simulink model "Tra_GearInfo"  (R2016b)
settings: configuration reference "CodeGenConfigSet" (kept outside this file)
values from neighbouring files (symbols this model uses):
  PT_stTraRevGear_C = Calibration.Parameter    [init_Tra_GearInfo.m]    (also in init_Tra_GearInfo_SIL.m = Simulink.Parameter)
  Tra_bStrtStopEnaDfl_C = Calibration.Parameter    [init_Tra_GearInfo.m]    (also in init_Tra_GearInfo_SIL.m = Simulink.Parameter)
  Tra_facN2NPT1_C = Calibration.Parameter    [init_Tra_GearInfo.m]    (also in init_Tra_GearInfo_SIL.m = Simulink.Parameter)
  Tra_facNPT1_C = Calibration.Parameter    [init_Tra_GearInfo.m]    (also in init_Tra_GearInfo_SIL.m = Simulink.Parameter)
  Tra_facV2NPT1_C = Calibration.Parameter    [init_Tra_GearInfo.m]    (also in init_Tra_GearInfo_SIL.m = Simulink.Parameter)
  Tra_GearWide_C = Calibration.Parameter    [init_Tra_GearInfo.m]    (also in init_Tra_GearInfo_SIL.m = Simulink.Parameter)
  Tra_nCrdShMin_C = Calibration.Parameter    [init_Tra_GearInfo.m]    (also in init_Tra_GearInfo_SIL.m = Simulink.Parameter)
  Tra_nEngMin_C = Calibration.Parameter    [init_Tra_GearInfo.m]    (also in init_Tra_GearInfo_SIL.m = Simulink.Parameter)
  Tra_numGearDfl1_C = Calibration.Parameter    [init_Tra_GearInfo.m]    (also in init_Tra_GearInfo_SIL.m = Simulink.Parameter)
  Tra_numGearDfl2_C = Calibration.Parameter    [init_Tra_GearInfo.m]    (also in init_Tra_GearInfo_SIL.m = Simulink.Parameter)
  Tra_numGearTable_CA = Calibration.Parameter    [init_Tra_GearInfo.m]    (also in init_Tra_GearInfo_SIL.m = Simulink.Parameter)
  Tra_rN2NGbxMax_C = Calibration.Parameter    [init_Tra_GearInfo.m]    (also in init_Tra_GearInfo_SIL.m = Simulink.Parameter)
  Tra_rN2NGbxMin_C = Calibration.Parameter    [init_Tra_GearInfo.m]    (also in init_Tra_GearInfo_SIL.m = Simulink.Parameter)
  Tra_rnFacCrdS_C = Calibration.Parameter    [init_Tra_GearInfo.m]    (also in init_Tra_GearInfo_SIL.m = Simulink.Parameter)
  Tra_rTransTable_CA = Calibration.Parameter    [init_Tra_GearInfo.m]    (also in init_Tra_GearInfo_SIL.m = Simulink.Parameter)
  Tra_rV2NDfl_C = Calibration.Parameter    [init_Tra_GearInfo.m]    (also in init_Tra_GearInfo_SIL.m = Simulink.Parameter)
  Tra_rV2NMax_C = Calibration.Parameter    [init_Tra_GearInfo.m]    (also in init_Tra_GearInfo_SIL.m = Simulink.Parameter)
  Tra_rV2NMin_C = Calibration.Parameter    [init_Tra_GearInfo.m]    (also in init_Tra_GearInfo_SIL.m = Simulink.Parameter)
  Tra_SumGear_C = Calibration.Parameter    [init_Tra_GearInfo.m]    (also in init_Tra_GearInfo_SIL.m = Simulink.Parameter)
  Tra_swtSrcCrdSSpdVal_C = Calibration.Parameter    [init_Tra_GearInfo.m]    (also in init_Tra_GearInfo_SIL.m = Simulink.Parameter)
undefined symbols (not defined in the file or in its folder): PT_TraType_State_conv, Switch_conv
libraries: CXLib x5
settings Model: PauseTimes=1  Creator=Colin  LastModifiedBy=bianxuyin
settings ConfigSetRef: SourceLocation=Base Workspace

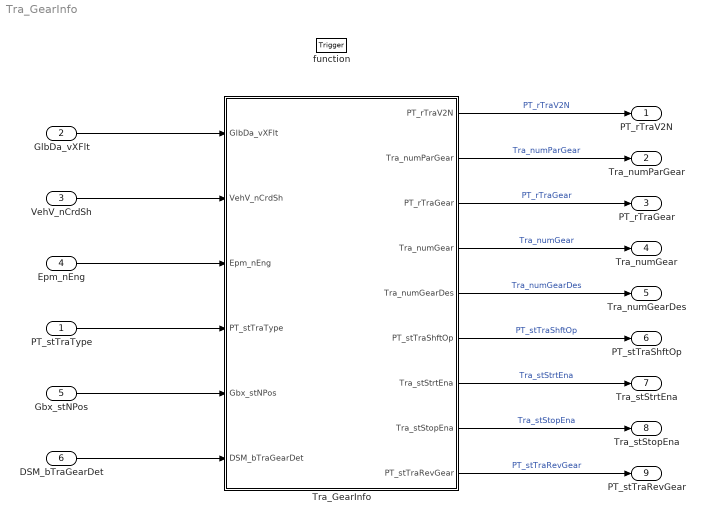
== system Tra_GearInfo ==
  PT_stTraType : Inport  Description=Current transmission type  OutDataTypeStr=Enum: PT_TraType_State_conv
  GlbDa_vXFlt : Inport  Tag=km/h  Description=Vehicle velocity filtered  Port=2  OutMin=0  OutMax=250  OutDataTypeStr=VehSpeed_km_h
  VehV_nCrdSh : Inport  Tag=rpm  Description=Cardan shaft speed  Port=3  OutMin=0  OutMax=6000  OutDataTypeStr=EngSpeed_rpm
  Epm_nEng : Inport  Tag=rpm  Description=Engine speed  Port=4  OutMin=0  OutMax=6000  OutDataTypeStr=EngSpeed_rpm
  Gbx_stNPos : Inport  Description=Gearbox neutral position status signal  Port=5  OutMin=0  OutMax=255  OutDataTypeStr=State_uint8
  DSM_bTraGearDet : Inport  Description=Fault Indicator of Gear Detect Function  Port=6  OutMin=0  OutMax=1  OutDataTypeStr=boolean
  function : TriggerPort  TriggerType=function-call  VariantControl=Variant
  Tra_GearInfo : Subsystem  RTWFcnName=Tra_GearInfo_Co  RTWFileName=Tra_GearInfo
      settings: RTWSystemCode=Nonreusable function  RTWFcnNameOpts=User specified  RTWFileNameOpts=User specified
  PT_rTraV2N : Outport  Tag=km/h/rpm  Description=Quotient of velocity and engine speed  OutMin=-0.32768  OutMax=0.32767  OutDataTypeStr=Tra_V2N_km_h_rpm
  Tra_numParGear : Outport  Description=Application parameter for gear number of the parameter gear of the transmission  Port=2  OutMin=-128  OutMax=127  OutDataTypeStr=Tra_num
  PT_rTraGear : Outport  Description=Current ratio for transmission  Port=3  OutMin=-100  OutMax=100  OutDataTypeStr=TransRatio
  Tra_numGear : Outport  Description=Current gear information  Port=4  OutMin=-128  OutMax=127  OutDataTypeStr=Tra_num
  Tra_numGearDes : Outport  Description=Application parameter for gear number of the destination gear of the transmission  Port=5  OutMin=-128  OutMax=127  OutDataTypeStr=Tra_num
  PT_stTraShftOp : Outport  Description=Status if shift operation is active  Port=6  OutMin=0  OutMax=1  OutDataTypeStr=boolean
  Tra_stStrtEna : Outport  Description=Enable start function  Port=7  OutMin=0  OutMax=1  OutDataTypeStr=boolean
  Tra_stStopEna : Outport  Description=Enable stop function  Port=8  OutMin=0  OutMax=1  OutDataTypeStr=boolean
  PT_stTraRevGear : Outport  Description=Status if reverse gear is selected  Port=9  OutMin=0  OutMax=1  OutDataTypeStr=boolean
  wires:
  Tra_GearInfo/2(Tra_numParGear) -> Tra_numParGear/1  "Tra_numParGear"
  Tra_GearInfo/3(PT_rTraGear) -> PT_rTraGear/1  "PT_rTraGear"
  Tra_GearInfo/4(Tra_numGear) -> Tra_numGear/1  "Tra_numGear"
  Tra_GearInfo/5(Tra_numGearDes) -> Tra_numGearDes/1  "Tra_numGearDes"
  Tra_GearInfo/6(PT_stTraShftOp) -> PT_stTraShftOp/1  "PT_stTraShftOp"
  Tra_GearInfo/7(Tra_stStrtEna) -> Tra_stStrtEna/1  "Tra_stStrtEna"
  Tra_GearInfo/8(Tra_stStopEna) -> Tra_stStopEna/1  "Tra_stStopEna"
  GlbDa_vXFlt/1 -> Tra_GearInfo/1(GlbDa_vXFlt)
  PT_stTraType/1 -> Tra_GearInfo/4(PT_stTraType)
  VehV_nCrdSh/1 -> Tra_GearInfo/2(VehV_nCrdSh)
  Epm_nEng/1 -> Tra_GearInfo/3(Epm_nEng)
  Gbx_stNPos/1 -> Tra_GearInfo/5(Gbx_stNPos)
  Tra_GearInfo/1(PT_rTraV2N) -> PT_rTraV2N/1  "PT_rTraV2N"
  DSM_bTraGearDet/1 -> Tra_GearInfo/6(DSM_bTraGearDet)
  Tra_GearInfo/9(PT_stTraRevGear) -> PT_stTraRevGear/1  "PT_stTraRevGear"

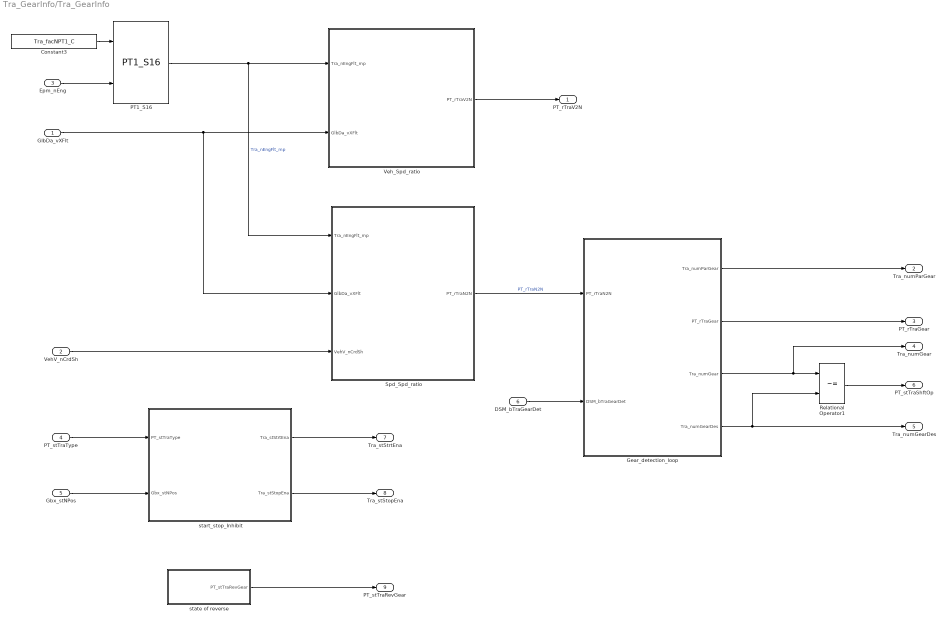
== system Tra_GearInfo/Tra_GearInfo ==
  GlbDa_vXFlt : Inport
  VehV_nCrdSh : Inport  Port=2
  Epm_nEng : Inport  Port=3
  PT_stTraType : Inport  Port=4
  Gbx_stNPos : Inport  Port=5
  DSM_bTraGearDet : Inport  Port=6
  Constant3 : Constant  RequirementInfo={} %GIDa_68e8745b_1911_4ff8_b2e8_39acb6395a61  Value=Tra_facNPT1_C  SampleTime=-1
  Gear_detection_loop : Subsystem
  PT1_S16 : CXLib/PT1_S16
  Relational Operator1 : RelationalOperator  Operator=~=  OutDataTypeStr=boolean  RndMeth=Simplest  InputSameDT=on
  Spd_Spd_ratio : Subsystem
  Veh_Spd_ratio : Subsystem
  start_stop_Inhibit : Subsystem
  state of reverse : Subsystem
  PT_rTraV2N : Outport
  Tra_numParGear : Outport  Port=2
  PT_rTraGear : Outport  Port=3
  Tra_numGear : Outport  Port=4
  Tra_numGearDes : Outport  Port=5
  PT_stTraShftOp : Outport  Port=6
  Tra_stStrtEna : Outport  Port=7
  Tra_stStopEna : Outport  Port=8
  PT_stTraRevGear : Outport  Port=9
  wires:
  Constant3/1 -> PT1_S16/1
  PT1_S16/1 -> Spd_Spd_ratio/1(Tra_nEngFlt_mp), Veh_Spd_ratio/1(Tra_nEngFlt_mp)  "Tra_nEngFlt_mp"
  Epm_nEng/1 -> PT1_S16/2
  Veh_Spd_ratio/1(PT_rTraV2N) -> PT_rTraV2N/1
  VehV_nCrdSh/1 -> Spd_Spd_ratio/3(VehV_nCrdSh)
  GlbDa_vXFlt/1 -> Spd_Spd_ratio/2(GlbDa_vXFlt), Veh_Spd_ratio/2(GlbDa_vXFlt)
  Gear_detection_loop/1(Tra_numParGear) -> Tra_numParGear/1
  Gear_detection_loop/2(PT_rTraGear) -> PT_rTraGear/1
  Gear_detection_loop/4(Tra_numGearDes) -> Relational Operator1/2, Tra_numGearDes/1
  Gear_detection_loop/3(Tra_numGear) -> Tra_numGear/1, Relational Operator1/1
  Spd_Spd_ratio/1(PT_rTraN2N) -> Gear_detection_loop/1(PT_rTraN2N)  "PT_rTraN2N"
  PT_stTraType/1 -> start_stop_Inhibit/1(PT_stTraType)
  Gbx_stNPos/1 -> start_stop_Inhibit/2(Gbx_stNPos)
  start_stop_Inhibit/1(Tra_stStrtEna) -> Tra_stStrtEna/1
  Relational Operator1/1 -> PT_stTraShftOp/1
  DSM_bTraGearDet/1 -> Gear_detection_loop/2(DSM_bTraGearDet)
  start_stop_Inhibit/2(Tra_stStopEna) -> Tra_stStopEna/1
  state of reverse/1(PT_stTraRevGear) -> PT_stTraRevGear/1

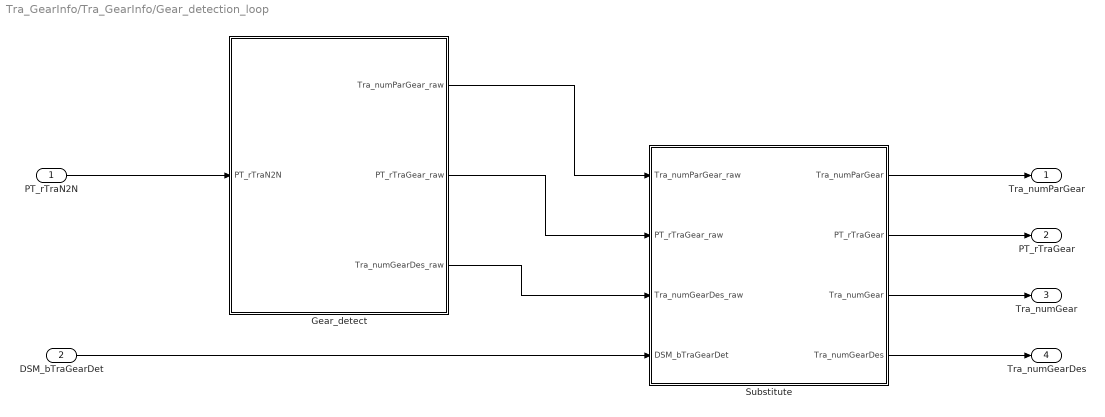
== system Tra_GearInfo/Tra_GearInfo/Gear_detection_loop ==
  PT_rTraN2N : Inport
  DSM_bTraGearDet : Inport  Port=2
  Gear_detect : Subsystem
  Substitute : Subsystem
  Tra_numParGear : Outport
  PT_rTraGear : Outport  Port=2
  Tra_numGear : Outport  Port=3
  Tra_numGearDes : Outport  Port=4
  wires:
  PT_rTraN2N/1 -> Gear_detect/1(PT_rTraN2N)
  Gear_detect/1(Tra_numParGear_raw) -> Substitute/1(Tra_numParGear_raw)
  Gear_detect/2(PT_rTraGear_raw) -> Substitute/2(PT_rTraGear_raw)
  Gear_detect/3(Tra_numGearDes_raw) -> Substitute/3(Tra_numGearDes_raw)
  DSM_bTraGearDet/1 -> Substitute/4(DSM_bTraGearDet)
  Substitute/1(Tra_numParGear) -> Tra_numParGear/1
  Substitute/2(PT_rTraGear) -> PT_rTraGear/1
  Substitute/3(Tra_numGear) -> Tra_numGear/1
  Substitute/4(Tra_numGearDes) -> Tra_numGearDes/1

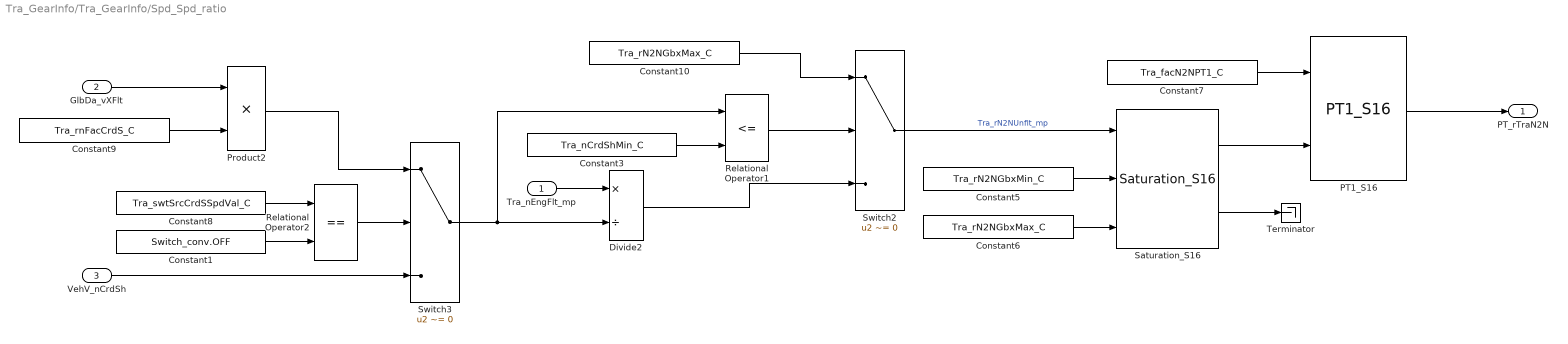
== system Tra_GearInfo/Tra_GearInfo/Spd_Spd_ratio ==
  Tra_nEngFlt_mp : Inport
  GlbDa_vXFlt : Inport  Port=2
  VehV_nCrdSh : Inport  Port=3
  Constant1 : Constant  Value=Switch_conv.OFF
  Constant10 : Constant  RequirementInfo={} %GIDa_6f34627e_a67b_41e5_bccd_7473a6215879  Value=Tra_rN2NGbxMax_C
  Constant3 : Constant  RequirementInfo={} %GIDa_5538a528_965c_4589_b0a7_730ad036b313  Value=Tra_nCrdShMin_C
  Constant5 : Constant  RequirementInfo={} %GIDa_afc6ce1b_0c3f_442d_8793_2f07f64178e4  Value=Tra_rN2NGbxMin_C
  Constant6 : Constant  RequirementInfo={} %GIDa_9ff4cd1f_23f8_4f85_9f7c_f07eb2272bcc  Value=Tra_rN2NGbxMax_C
  Constant7 : Constant  RequirementInfo={} %GIDa_94a5a4cc_14d9_42df_a91a_5d387bca77db  Value=Tra_facN2NPT1_C
  Constant8 : Constant  RequirementInfo={} %GIDa_6b600eae_0818_4397_83da_58a64cbb6d28  Value=Tra_swtSrcCrdSSpdVal_C
  Constant9 : Constant  RequirementInfo={} %GIDa_ceae6799_0a24_4591_adf3_94fda113d9ac  Value=Tra_rnFacCrdS_C
  Divide2 : Product  Inputs=*/  OutDataTypeStr=Inherit: Inherit via back propagation  SaturateOnIntegerOverflow=on
  PT1_S16 : CXLib/PT1_S16
  Product2 : Product  OutDataTypeStr=EngSpeed_rpm  SaturateOnIntegerOverflow=on
  Relational Operator1 : RelationalOperator  Operator=<=  OutDataTypeStr=boolean  RndMeth=Simplest  InputSameDT=on
  Relational Operator2 : RelationalOperator  Operator===  OutDataTypeStr=boolean  RndMeth=Simplest  InputSameDT=on
  Saturation_S16 : CXLib/Saturation_S16
  Switch2 : Switch  Criteria=u2 ~= 0  InputSameDT=on
  Switch3 : Switch  Criteria=u2 ~= 0  InputSameDT=on
  Terminator : Terminator
  PT_rTraN2N : Outport
  wires:
  Constant5/1 -> Saturation_S16/2
  Constant3/1 -> Relational Operator1/2
  Constant6/1 -> Saturation_S16/3
  Saturation_S16/2 -> Terminator/1
  PT1_S16/1 -> PT_rTraN2N/1
  Saturation_S16/1 -> PT1_S16/2
  Constant7/1 -> PT1_S16/1
  Product2/1 -> Switch3/1
  Constant9/1 -> Product2/2
  Switch3/1 -> Relational Operator1/1, Divide2/2
  Divide2/1 -> Switch2/3
  Relational Operator1/1 -> Switch2/2
  Constant10/1 -> Switch2/1
  Switch2/1 -> Saturation_S16/1  "Tra_rN2NUnflt_mp"
  Tra_nEngFlt_mp/1 -> Divide2/1
  GlbDa_vXFlt/1 -> Product2/1
  VehV_nCrdSh/1 -> Switch3/3
  Relational Operator2/1 -> Switch3/2
  Constant1/1 -> Relational Operator2/2
  Constant8/1 -> Relational Operator2/1

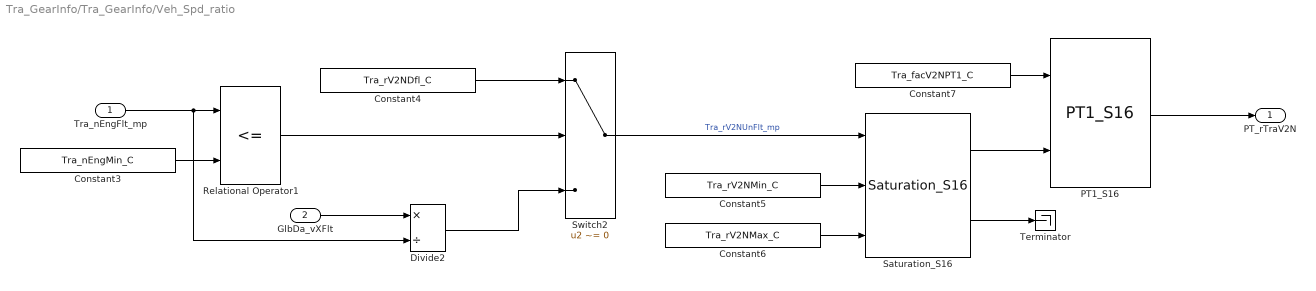
== system Tra_GearInfo/Tra_GearInfo/Veh_Spd_ratio ==
  Tra_nEngFlt_mp : Inport
  GlbDa_vXFlt : Inport  Port=2
  Constant3 : Constant  RequirementInfo={} %GIDa_0ea41357_8063_45a9_a77a_64950543f60f  Value=Tra_nEngMin_C
  Constant4 : Constant  RequirementInfo={} %GIDa_6683fc9c_f2a5_4281_9c47_91a20911e949  Value=Tra_rV2NDfl_C
  Constant5 : Constant  RequirementInfo={} %GIDa_5f74a71a_760f_4d90_b253_e16e90e61e58  Value=Tra_rV2NMin_C
  Constant6 : Constant  RequirementInfo={} %GIDa_e28cada3_7ccc_4ace_b1a6_ef9bbdcca018  Value=Tra_rV2NMax_C
  Constant7 : Constant  RequirementInfo={} %GIDa_7cf28180_be86_401f_bbee_9342c25283e2  Value=Tra_facV2NPT1_C
  Divide2 : Product  Inputs=*/  OutDataTypeStr=Tra_V2N_km_h_rpm
  PT1_S16 : CXLib/PT1_S16
  Relational Operator1 : RelationalOperator  Operator=<=  OutDataTypeStr=boolean  RndMeth=Simplest  InputSameDT=on
  Saturation_S16 : CXLib/Saturation_S16
  Switch2 : Switch  Criteria=u2 ~= 0  InputSameDT=on
  Terminator : Terminator
  PT_rTraV2N : Outport
  wires:
  Relational Operator1/1 -> Switch2/2
  Constant3/1 -> Relational Operator1/2
  Tra_nEngFlt_mp/1 -> Divide2/2, Relational Operator1/1
  Constant6/1 -> Saturation_S16/3
  Saturation_S16/2 -> Terminator/1
  Constant5/1 -> Saturation_S16/2
  Divide2/1 -> Switch2/3
  Constant4/1 -> Switch2/1
  Switch2/1 -> Saturation_S16/1  "Tra_rV2NUnFlt_mp"
  PT1_S16/1 -> PT_rTraV2N/1
  Saturation_S16/1 -> PT1_S16/2
  Constant7/1 -> PT1_S16/1
  GlbDa_vXFlt/1 -> Divide2/1

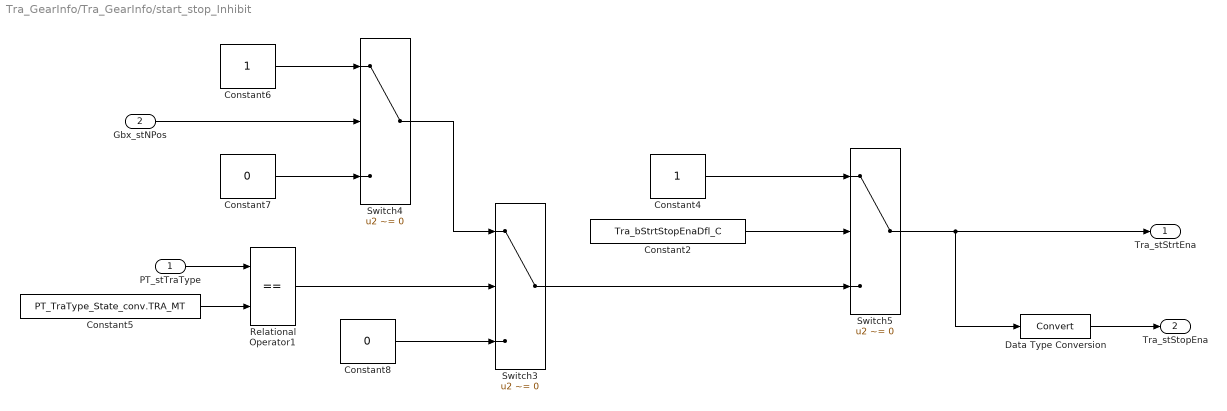
== system Tra_GearInfo/Tra_GearInfo/start_stop_Inhibit ==
  PT_stTraType : Inport
  Gbx_stNPos : Inport  Port=2
  Constant2 : Constant  RequirementInfo={} %GIDa_1bf9b28b_75ea_4a97_98e6_f79f35991fee  Value=Tra_bStrtStopEnaDfl_C
  Constant4 : Constant  RequirementInfo={} %GIDa_d4fd0d66_3232_4b6d_9285_aae7ee49d272  OutDataTypeStr=boolean
  Constant5 : Constant  RequirementInfo={} %GIDa_0b0c96fa_d8ca_4914_a52e_fa2a4c075e46  Value=PT_TraType_State_conv.TRA_MT
  Constant6 : Constant  RequirementInfo={} %GIDa_1d15985e_156c_46b3_90ae_da8f21aeea05  OutDataTypeStr=boolean
  Constant7 : Constant  RequirementInfo={} %GIDa_ec4582e0_b9c2_48c9_a922_0b8eaa2522c1  Value=0  OutDataTypeStr=boolean
  Constant8 : Constant  RequirementInfo={} %GIDa_577e0d94_e6f9_475f_ab73_b6aca9ed7e20  Value=0  OutDataTypeStr=boolean
  Data Type Conversion : DataTypeConversion
  Relational Operator1 : RelationalOperator  Operator===  OutDataTypeStr=boolean  RndMeth=Simplest  InputSameDT=on
  Switch3 : Switch  Criteria=u2 ~= 0  InputSameDT=on
  Switch4 : Switch  Criteria=u2 ~= 0  InputSameDT=on
  Switch5 : Switch  Criteria=u2 ~= 0  InputSameDT=on
  Tra_stStrtEna : Outport
  Tra_stStopEna : Outport  Port=2
  wires:
  Constant6/1 -> Switch4/1
  Relational Operator1/1 -> Switch3/2
  Constant8/1 -> Switch3/3
  Switch3/1 -> Switch5/3
  Constant4/1 -> Switch5/1
  Constant2/1 -> Switch5/2
  Constant5/1 -> Relational Operator1/2
  Constant7/1 -> Switch4/3
  Gbx_stNPos/1 -> Switch4/2
  Switch4/1 -> Switch3/1
  PT_stTraType/1 -> Relational Operator1/1
  Switch5/1 -> Data Type Conversion/1, Tra_stStrtEna/1
  Data Type Conversion/1 -> Tra_stStopEna/1

== system Tra_GearInfo/Tra_GearInfo/state of reverse ==
  Constant : Constant  Value=PT_stTraRevGear_C
  Data Type Conversion : DataTypeConversion
  PT_stTraRevGear : Outport
  wires:
  Data Type Conversion/1 -> PT_stTraRevGear/1
  Constant/1 -> Data Type Conversion/1

== system Tra_GearInfo/Tra_GearInfo/Gear_detection_loop/Gear_detect ==
  PT_rTraN2N : Inport
  Constant : Constant  Value=0  OutDataTypeStr=Tra_num
  Constant1 : Constant  Value=true  OutDataTypeStr=boolean
  While Iterator Subsystem : Subsystem  TreatAsAtomicUnit=on
  Tra_numParGear_raw : Outport
  PT_rTraGear_raw : Outport  Port=2
  Tra_numGearDes_raw : Outport  Port=3
  wires:
  Constant/1 -> Tra_numGearDes_raw/1
  PT_rTraN2N/1 -> While Iterator Subsystem/1(PT_rTraN2N)
  Constant1/1 -> While Iterator Subsystem/2(IC)
  While Iterator Subsystem/1(Tra_numParGear) -> Tra_numParGear_raw/1
  While Iterator Subsystem/2(PT_rTraGear) -> PT_rTraGear_raw/1

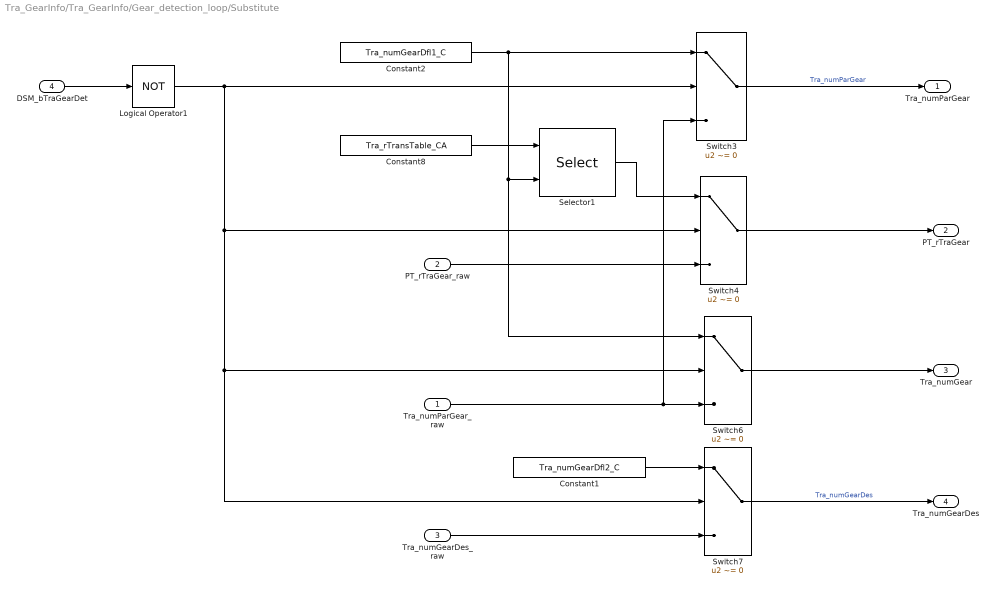
== system Tra_GearInfo/Tra_GearInfo/Gear_detection_loop/Substitute ==
  Tra_numParGear_raw : Inport
  PT_rTraGear_raw : Inport  Port=2
  Tra_numGearDes_raw : Inport  Port=3
  DSM_bTraGearDet : Inport  Port=4
  Constant1 : Constant  RequirementInfo={} %GIDa_abaaa14e_1b52_4b72_9892_7989d78ea5be  Value=Tra_numGearDfl2_C
  Constant2 : Constant  RequirementInfo={} %GIDa_3784fce9_4740_4465_a8b9_99d9112f29e3  Value=Tra_numGearDfl1_C
  Constant8 : Constant  RequirementInfo={} %GIDa_bc77505f_8ff4_4c5c_a4a3_7568016e4e8d  Value=Tra_rTransTable_CA
  Logical Operator1 : Logic  Operator=NOT  AllPortsSameDT=off  OutDataTypeStr=boolean
  Selector1 : Selector  IndexMode=Zero-based  InputPortWidth=26  IndexOptions=Index vector (port)  Indices=[1 3]  OutputSizes=1
  Switch{3..4,6..7} (4 alike) : Switch  Criteria=u2 ~= 0  InputSameDT=on
  Tra_numParGear : Outport
  PT_rTraGear : Outport  Port=2
  Tra_numGear : Outport  Port=3
  Tra_numGearDes : Outport  Port=4
  wires:
  Selector1/1 -> Switch4/1
  Constant2/1 -> Switch3/1, Switch6/1, Selector1/2
  Constant1/1 -> Switch7/1
  Switch3/1 -> Tra_numParGear/1  "Tra_numParGear"
  Switch4/1 -> PT_rTraGear/1
  Switch6/1 -> Tra_numGear/1
  Tra_numParGear_raw/1 -> Switch3/3, Switch6/3
  DSM_bTraGearDet/1 -> Logical Operator1/1
  Switch7/1 -> Tra_numGearDes/1  "Tra_numGearDes"
  PT_rTraGear_raw/1 -> Switch4/3
  Tra_numGearDes_raw/1 -> Switch7/3
  Logical Operator1/1 -> Switch7/2, Switch6/2, Switch4/2, Switch3/2
  Constant8/1 -> Selector1/1

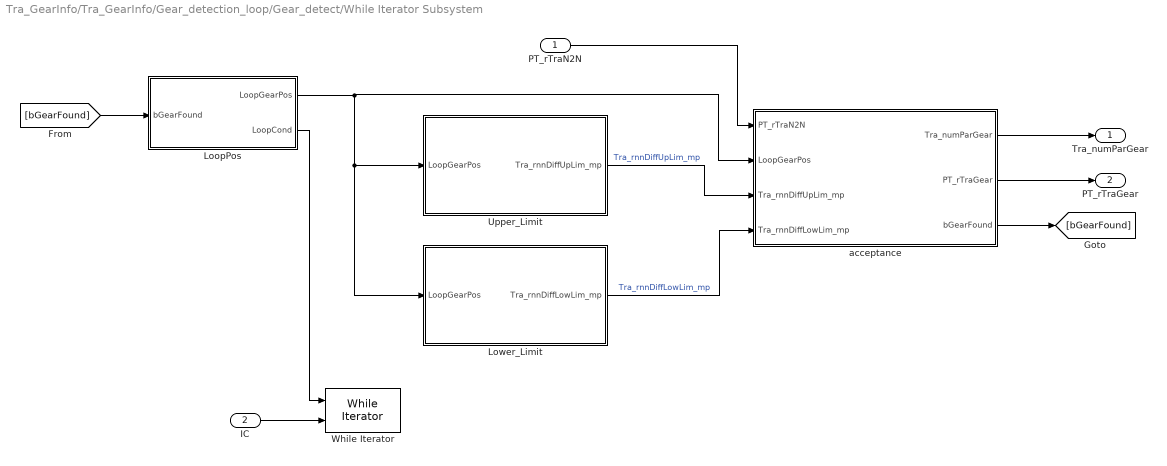
== system Tra_GearInfo/Tra_GearInfo/Gear_detection_loop/Gear_detect/While Iterator Subsystem ==
  PT_rTraN2N : Inport
  IC : Inport  Port=2
  LoopPos : Subsystem
  Lower_Limit : Subsystem
      settings: MinAlgLoopOccurrences=on  RTWSystemCode=Nonreusable function
  Upper_Limit : Subsystem
      settings: MinAlgLoopOccurrences=on  RTWSystemCode=Nonreusable function
  While Iterator : WhileIterator  MaxIters=26  ResetStates=reset
  acceptance : Subsystem
  Tra_numParGear : Outport
  PT_rTraGear : Outport  Port=2
  wires:
  Lower_Limit/1(Tra_rnnDiffLowLim_mp) -> acceptance/4(Tra_rnnDiffLowLim_mp)  "Tra_rnnDiffLowLim_mp"
  Upper_Limit/1(Tra_rnnDiffUpLim_mp) -> acceptance/3(Tra_rnnDiffUpLim_mp)  "Tra_rnnDiffUpLim_mp"
  PT_rTraN2N/1 -> acceptance/1(PT_rTraN2N)
  LoopPos/1(LoopGearPos) -> acceptance/2(LoopGearPos), Lower_Limit/1(LoopGearPos), Upper_Limit/1(LoopGearPos)
  acceptance/3(bGearFound) -> [bGearFound]
  IC/1 -> While Iterator/2
  LoopPos/2(LoopCond) -> While Iterator/1
  [bGearFound] -> LoopPos/1(bGearFound)
  acceptance/1(Tra_numParGear) -> Tra_numParGear/1
  acceptance/2(PT_rTraGear) -> PT_rTraGear/1

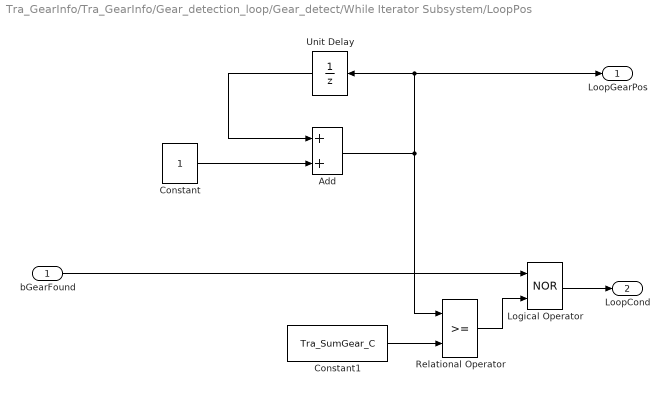
== system Tra_GearInfo/Tra_GearInfo/Gear_detection_loop/Gear_detect/While Iterator Subsystem/LoopPos ==
  bGearFound : Inport
  Add : Sum
  Constant : Constant  OutDataTypeStr=Tra_num
  Constant1 : Constant  Value=Tra_SumGear_C
  Logical Operator : Logic  Operator=NOR  AllPortsSameDT=off  OutDataTypeStr=boolean
  Relational Operator : RelationalOperator  OutDataTypeStr=boolean  RndMeth=Simplest  InputSameDT=on
  Unit Delay : UnitDelay  SampleTime=-1
      settings: AttributesFormatString=InitialValue=%<InitialCondition>
  LoopGearPos : Outport
  LoopCond : Outport  Port=2
  wires:
  Constant/1 -> Add/2
  Unit Delay/1 -> Add/1
  Add/1 -> Relational Operator/1, Unit Delay/1, LoopGearPos/1
  bGearFound/1 -> Logical Operator/1
  Relational Operator/1 -> Logical Operator/2
  Constant1/1 -> Relational Operator/2
  Logical Operator/1 -> LoopCond/1

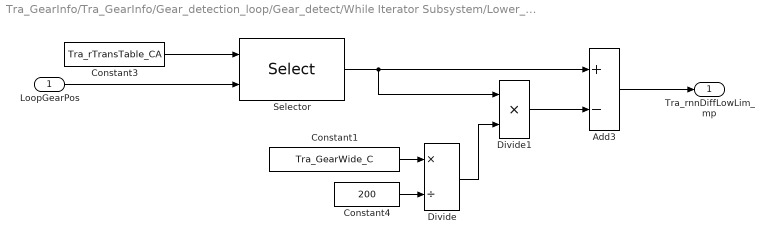
== system Tra_GearInfo/Tra_GearInfo/Gear_detection_loop/Gear_detect/While Iterator Subsystem/Lower_Limit ==
  LoopGearPos : Inport  OutMin=0  OutMax=25
  Add3 : Sum  Inputs=+-  InputSameDT=on
  Constant1 : Constant  RequirementInfo={} %GIDa_061c3916_d79c_4568_919c_4bbcfe29e0af  Value=Tra_GearWide_C
  Constant3 : Constant  Value=Tra_rTransTable_CA
  Constant4 : Constant  RequirementInfo={} %GIDa_fa577c3e_2c55_430a_9fa9_c4eca1af02d0  Value=200  OutDataTypeStr=uint8
  Divide : Product  Inputs=*/  OutDataTypeStr=Fact1
  Divide1 : Product  Inputs=**  OutDataTypeStr=Inherit: Inherit via back propagation
  Selector : Selector  IndexMode=Zero-based  InputPortWidth=26  IndexOptions=Index vector (port)  Indices=[1 3]  OutputSizes=1
  Tra_rnnDiffLowLim_mp : Outport
  wires:
  Constant1/1 -> Divide/1
  Constant4/1 -> Divide/2
  Divide/1 -> Divide1/2
  Divide1/1 -> Add3/2
  Add3/1 -> Tra_rnnDiffLowLim_mp/1
  Selector/1 -> Divide1/1, Add3/1
  Constant3/1 -> Selector/1
  LoopGearPos/1 -> Selector/2

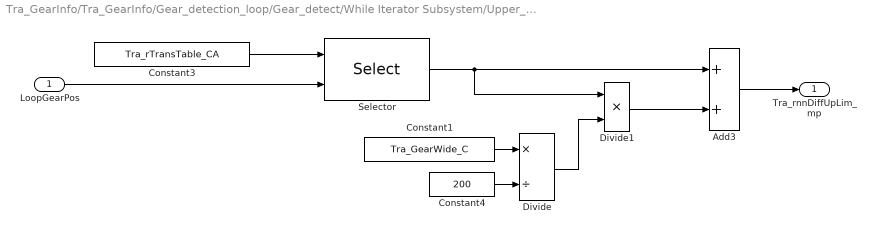
== system Tra_GearInfo/Tra_GearInfo/Gear_detection_loop/Gear_detect/While Iterator Subsystem/Upper_Limit ==
  LoopGearPos : Inport  OutMin=0  OutMax=25
  Add3 : Sum  InputSameDT=on
  Constant1 : Constant  RequirementInfo={} %GIDa_c587f4ae_2db6_46bd_b920_d4b71c2fff0f  Value=Tra_GearWide_C
  Constant3 : Constant  Value=Tra_rTransTable_CA
  Constant4 : Constant  RequirementInfo={} %GIDa_a013eb5b_6f2d_4ebc_a867_495d4abc60cd  Value=200  OutDataTypeStr=uint8
  Divide : Product  Inputs=*/  OutDataTypeStr=Fact1
  Divide1 : Product  Inputs=**  OutDataTypeStr=Inherit: Inherit via back propagation
  Selector : Selector  IndexMode=Zero-based  InputPortWidth=26  IndexOptions=Index vector (port)  Indices=[1 3]  OutputSizes=1
  Tra_rnnDiffUpLim_mp : Outport
  wires:
  Constant1/1 -> Divide/1
  Constant4/1 -> Divide/2
  Divide/1 -> Divide1/2
  Divide1/1 -> Add3/2
  Add3/1 -> Tra_rnnDiffUpLim_mp/1
  Selector/1 -> Divide1/1, Add3/1
  Constant3/1 -> Selector/1
  LoopGearPos/1 -> Selector/2

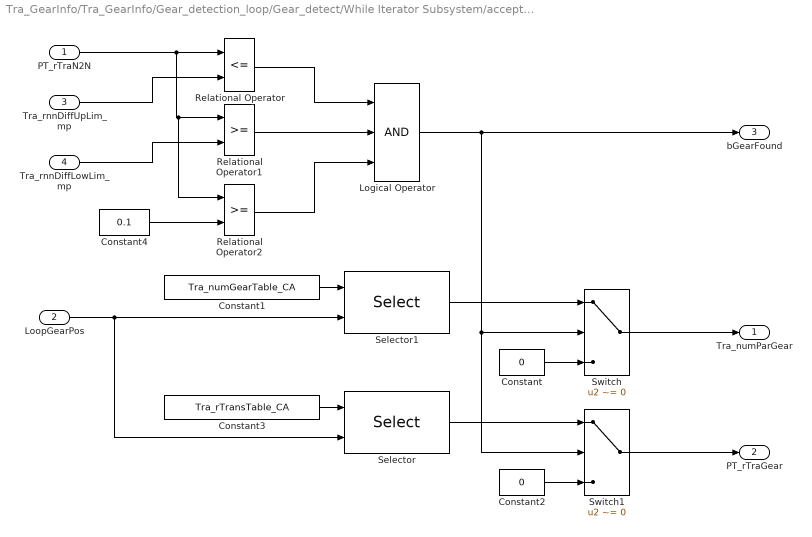
== system Tra_GearInfo/Tra_GearInfo/Gear_detection_loop/Gear_detect/While Iterator Subsystem/acceptance ==
  PT_rTraN2N : Inport
  LoopGearPos : Inport  Port=2
  Tra_rnnDiffUpLim_mp : Inport  Port=3
  Tra_rnnDiffLowLim_mp : Inport  Port=4
  Constant : Constant  Value=0  OutDataTypeStr=Tra_num
  Constant1 : Constant  Value=Tra_numGearTable_CA
  Constant2 : Constant  Value=0  OutDataTypeStr=TransRatio
  Constant3 : Constant  Value=Tra_rTransTable_CA
  Constant4 : Constant  Value=0.1  OutDataTypeStr=TransRatio
  Logical Operator : Logic  Inputs=3  AllPortsSameDT=off  OutDataTypeStr=boolean
  Relational Operator : RelationalOperator  Operator=<=  OutDataTypeStr=boolean  RndMeth=Simplest
  Relational Operator1 : RelationalOperator  OutDataTypeStr=boolean  RndMeth=Simplest
  Relational Operator2 : RelationalOperator  OutDataTypeStr=boolean  RndMeth=Simplest
  Selector : Selector  IndexMode=Zero-based  InputPortWidth=26  IndexOptions=Index vector (port)  Indices=[1 3]  OutputSizes=1
  Selector1 : Selector  IndexMode=Zero-based  InputPortWidth=26  IndexOptions=Index vector (port)  Indices=[1 3]  OutputSizes=1
  Switch : Switch  Criteria=u2 ~= 0  InputSameDT=on
  Switch1 : Switch  Criteria=u2 ~= 0  InputSameDT=on
  Tra_numParGear : Outport
  PT_rTraGear : Outport  Port=2
  bGearFound : Outport  Port=3
  wires:
  PT_rTraN2N/1 -> Relational Operator2/1, Relational Operator1/1, Relational Operator/1
  Tra_rnnDiffUpLim_mp/1 -> Relational Operator/2
  Tra_rnnDiffLowLim_mp/1 -> Relational Operator1/2
  Relational Operator/1 -> Logical Operator/1
  Relational Operator1/1 -> Logical Operator/2
  Switch/1 -> Tra_numParGear/1
  Constant/1 -> Switch/3
  Logical Operator/1 -> Switch1/2, Switch/2, bGearFound/1
  LoopGearPos/1 -> Selector/2, Selector1/2
  Constant3/1 -> Selector/1
  Constant1/1 -> Selector1/1
  Selector1/1 -> Switch/1
  Switch1/1 -> PT_rTraGear/1
  Constant2/1 -> Switch1/3
  Selector/1 -> Switch1/1
  Constant4/1 -> Relational Operator2/2
  Relational Operator2/1 -> Logical Operator/3
